simulink subsystem "ControladorBA"  (R2022b)
settings: Solver=VariableStepAuto  StartTime=0.0  StopTime=10.0  RelTol=1e-3
settings Model: Creator=dar.io  LastModifiedBy=dar.io

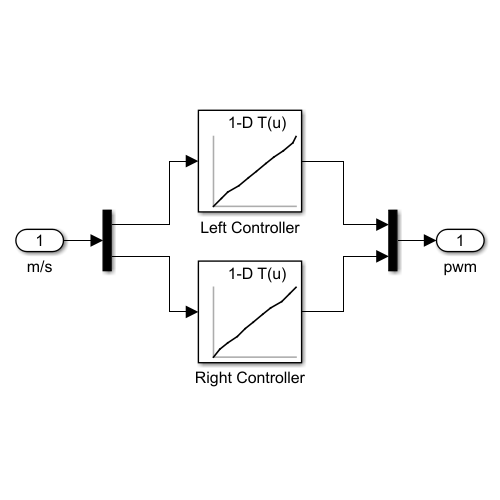
[thumbnail: Simulink's stored preview of the top-level diagram]
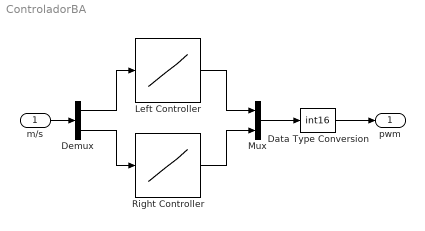
== system ControladorBA ==
  m/s : Inport
  Data Type Conversion : DataTypeConversion  OutDataTypeStr=int16  SaturateOnIntegerOverflow=off  RndMeth=Floor
  Demux : Demux  Outputs=2
  Left Controller : Lookup_n-D  NumberOfTableDimensions=1  BreakpointsForDimension1=[-0.494312286376953 -0.400794982910156 -0.320632934570313 -0.200393676757813 -0.0935134887695313 0 0.120246887207031 0.213752746582031 0.320640563964844 0.427513122558594 0.467594146728516]  Table=[-255 -200 -150 -100 -50 0 50 100 150 200 255]  InternalRulePriority=Speed  RndMeth=Simplest
  Mux : Mux  Inputs=2
  Right Controller : Lookup_n-D  NumberOfTableDimensions=1  BreakpointsForDimension1=[-0.48095703125 -0.400787353515625 -0.307273864746094 -0.187042236328125 -0.0935211181640625 0 0.1202392578125 0.213752746582031 0.34735107421875 0.440872192382813 0.521034240722656]  Table=[-255 -200 -150 -100 -50 0 50 100 150 200 255]  InternalRulePriority=Speed  RndMeth=Simplest
  pwm : Outport  OutDataTypeStr=int16
  wires:
  Demux/1 -> Left Controller/1
  Left Controller/1 -> Mux/1
  Demux/2 -> Right Controller/1
  Right Controller/1 -> Mux/2
  m/s/1 -> Demux/1
  Mux/1 -> Data Type Conversion/1
  Data Type Conversion/1 -> pwm/1
